simulink model "IEEE9_case"  (R2024b)
settings: Solver=FixedStepAuto  StartTime=0  StopTime=5  FixedStep=1e-7  RelTol=1e-3
values from neighbouring files (symbols this model uses):
  SG_D_1_D = 0.01056    [IEEE9_case_parameters.m]    (also in case1_parameters.m; case2_parameters.m; case3_parameters.m; case4_parameters.m)
  SG_D_1_EnableSaturation = 0    [IEEE9_case_parameters.m]    (also in case1_parameters.m; case2_parameters.m; case3_parameters.m; case4_parameters.m)
  SG_D_1_f0 = 60    [IEEE9_case_parameters.m]    (also in case1_parameters.m; case2_parameters.m; case3_parameters.m; case4_parameters.m)
  SG_D_1_H = 7.5    [IEEE9_case_parameters.m]    (also in case1_parameters.m; case2_parameters.m; case3_parameters.m; case4_parameters.m)
  SG_D_1_K_A = 20    [IEEE9_case_parameters.m]    (also in case1_parameters.m; case2_parameters.m; case3_parameters.m; case4_parameters.m)
  SG_D_1_K_E = 1.000000e+1    (= 10)    [IEEE9_case_parameters.m]    (also in case1_parameters.m; case2_parameters.m; case3_parameters.m; case4_parameters.m)
  SG_D_1_K_F = 2.363    [IEEE9_case_parameters.m]    (also in case1_parameters.m; case2_parameters.m; case3_parameters.m; case4_parameters.m)
  SG_D_1_K_s = 0.5    [IEEE9_case_parameters.m]    (also in case1_parameters.m = 5; case2_parameters.m = 5; case3_parameters.m = 5; case4_parameters.m = 5)
  SG_D_1_R_a = 0.001088    [IEEE9_case_parameters.m]    (also in case1_parameters.m; case2_parameters.m; case3_parameters.m; case4_parameters.m)
  SG_D_1_S_A = 1    [IEEE9_case_parameters.m]    (also in case1_parameters.m; case2_parameters.m; case3_parameters.m; case4_parameters.m)
  SG_D_1_S_B = 0.103    [IEEE9_case_parameters.m]    (also in case1_parameters.m; case2_parameters.m; case3_parameters.m; case4_parameters.m)
  SG_D_1_S_N = 10.659857    [IEEE9_case_parameters.m]    (also in case1_parameters.m; case2_parameters.m; case3_parameters.m; case4_parameters.m)
  SG_D_1_SpeedPara = 200    [IEEE9_case_parameters.m]    (also in case1_parameters.m; case2_parameters.m; case3_parameters.m; case4_parameters.m)
  SG_D_1_T_0 = 0.720173    [IEEE9_case_parameters.m]    (also in case1_parameters.m = 0.755522; case2_parameters.m = 0.808931; case3_parameters.m = 0.869402; case4_parameters.m = 0.729316)
  SG_D_1_T_1 = 0.3    [IEEE9_case_parameters.m]    (also in case1_parameters.m; case2_parameters.m; case3_parameters.m; case4_parameters.m)
  SG_D_1_T_2 = 0.05    [IEEE9_case_parameters.m]    (also in case1_parameters.m; case2_parameters.m; case3_parameters.m; case4_parameters.m)
  SG_D_1_T_3 = 0.02    [IEEE9_case_parameters.m]    (also in case1_parameters.m; case2_parameters.m; case3_parameters.m; case4_parameters.m)
  SG_D_1_T_4 = 0.005    [IEEE9_case_parameters.m]    (also in case1_parameters.m; case2_parameters.m; case3_parameters.m; case4_parameters.m)
  SG_D_1_T_A = 0.02    [IEEE9_case_parameters.m]    (also in case1_parameters.m; case2_parameters.m; case3_parameters.m; case4_parameters.m)
  SG_D_1_T_dd = 8.000000e+0    (= 8)    [IEEE9_case_parameters.m]    (also in case1_parameters.m; case2_parameters.m; case3_parameters.m; case4_parameters.m)
  SG_D_1_T_ddd = 0.04    [IEEE9_case_parameters.m]    (also in case1_parameters.m; case2_parameters.m; case3_parameters.m; case4_parameters.m)
  SG_D_1_T_E = 0.314    [IEEE9_case_parameters.m]    (also in case1_parameters.m; case2_parameters.m; case3_parameters.m; case4_parameters.m)
  SG_D_1_T_F = 0.35    [IEEE9_case_parameters.m]    (also in case1_parameters.m; case2_parameters.m; case3_parameters.m; case4_parameters.m)
  SG_D_1_T_qd = 0.8    [IEEE9_case_parameters.m]    (also in case1_parameters.m; case2_parameters.m; case3_parameters.m; case4_parameters.m)
  SG_D_1_T_qdd = 0.02    [IEEE9_case_parameters.m]    (also in case1_parameters.m; case2_parameters.m; case3_parameters.m; case4_parameters.m)
  SG_D_1_T_speed = 0.1    [IEEE9_case_parameters.m]    (also in case1_parameters.m = 200; case2_parameters.m = 200; case3_parameters.m = 200; case4_parameters.m = 200)
  SG_D_1_T_w = 0.5    [IEEE9_case_parameters.m]    (also in case1_parameters.m; case2_parameters.m; case3_parameters.m; case4_parameters.m)
  SG_D_1_V_ref = 1.990276    [IEEE9_case_parameters.m]    (also in case1_parameters.m = 2.042296; case2_parameters.m = 2.051388; case3_parameters.m = 2.089584; case4_parameters.m = 2.01845)
  SG_D_1_w_ref = 376.991118    [IEEE9_case_parameters.m]    (also in case1_parameters.m; case2_parameters.m; case3_parameters.m; case4_parameters.m)
  SG_D_1_wb = 6.000000e+1    (= 60)    [IEEE9_case_parameters.m]    (also in case1_parameters.m; case2_parameters.m; case3_parameters.m; case4_parameters.m)
  SG_D_1_x_d = 1.9    [IEEE9_case_parameters.m]    (also in case1_parameters.m; case2_parameters.m; case3_parameters.m; case4_parameters.m)
  SG_D_1_x_dd = 0.302    [IEEE9_case_parameters.m]    (also in case1_parameters.m; case2_parameters.m; case3_parameters.m; case4_parameters.m)
  SG_D_1_x_ddd = 0.204    [IEEE9_case_parameters.m]    (also in case1_parameters.m; case2_parameters.m; case3_parameters.m; case4_parameters.m)
  SG_D_1_x_l = 0.05    [IEEE9_case_parameters.m]    (also in case1_parameters.m; case2_parameters.m; case3_parameters.m; case4_parameters.m)
  SG_D_1_x_q = 1.3    [IEEE9_case_parameters.m]    (also in case1_parameters.m; case2_parameters.m; case3_parameters.m; case4_parameters.m)
  SG_D_1_x_qd = 0.5    [IEEE9_case_parameters.m]    (also in case1_parameters.m; case2_parameters.m; case3_parameters.m; case4_parameters.m)
  SG_D_1_x_qdd = 0.3    [IEEE9_case_parameters.m]    (also in case1_parameters.m; case2_parameters.m; case3_parameters.m; case4_parameters.m)
  SG_D_2_D = 0.02    [IEEE9_case_parameters.m]    (also in case1_parameters.m; case2_parameters.m; case3_parameters.m; case4_parameters.m)
  SG_D_2_EnableSaturation = 0    [IEEE9_case_parameters.m]    (also in case1_parameters.m; case2_parameters.m; case3_parameters.m; case4_parameters.m)
  SG_D_2_f0 = 60    [IEEE9_case_parameters.m]    (also in case1_parameters.m; case2_parameters.m; case3_parameters.m; case4_parameters.m)
  SG_D_2_H = 8.000000e+0    (= 8)    [IEEE9_case_parameters.m]    (also in case1_parameters.m; case2_parameters.m; case3_parameters.m; case4_parameters.m)
  SG_D_2_K_A = 20    [IEEE9_case_parameters.m]    (also in case1_parameters.m; case2_parameters.m; case3_parameters.m; case4_parameters.m)
  SG_D_2_K_E = 1.000000e+1    (= 10)    [IEEE9_case_parameters.m]    (also in case1_parameters.m; case2_parameters.m; case3_parameters.m; case4_parameters.m)
  SG_D_2_K_F = 2.363    [IEEE9_case_parameters.m]    (also in case1_parameters.m; case2_parameters.m; case3_parameters.m; case4_parameters.m)
  SG_D_2_K_s = 0.5    [IEEE9_case_parameters.m]    (also in case1_parameters.m = 4; case2_parameters.m = 4; case3_parameters.m = 4; case4_parameters.m = 4)
  SG_D_2_R_a = 0.001088    [IEEE9_case_parameters.m]    (also in case1_parameters.m; case2_parameters.m; case3_parameters.m; case4_parameters.m)
  SG_D_2_S_A = 1    [IEEE9_case_parameters.m]    (also in case1_parameters.m; case2_parameters.m; case3_parameters.m; case4_parameters.m)
  SG_D_2_S_B = 0.103    [IEEE9_case_parameters.m]    (also in case1_parameters.m; case2_parameters.m; case3_parameters.m; case4_parameters.m)
  SG_D_2_S_N = 10.659857    [IEEE9_case_parameters.m]    (also in case1_parameters.m; case2_parameters.m; case3_parameters.m; case4_parameters.m)
  SG_D_2_SpeedPara = 200    [IEEE9_case_parameters.m]    (also in case1_parameters.m; case2_parameters.m; case3_parameters.m; case4_parameters.m)
  SG_D_2_T_0 = 1.632913    [IEEE9_case_parameters.m]    (also in case1_parameters.m = 1.632925; case2_parameters.m = 1.632915; case3_parameters.m = 1.632914; case4_parameters.m = 1.632927)
  SG_D_2_T_1 = 0.2    [IEEE9_case_parameters.m]    (also in case1_parameters.m; case2_parameters.m; case3_parameters.m; case4_parameters.m)
  SG_D_2_T_2 = 0.05    [IEEE9_case_parameters.m]    (also in case1_parameters.m; case2_parameters.m; case3_parameters.m; case4_parameters.m)
  SG_D_2_T_3 = 0.02    [IEEE9_case_parameters.m]    (also in case1_parameters.m; case2_parameters.m; case3_parameters.m; case4_parameters.m)
  SG_D_2_T_4 = 0.005    [IEEE9_case_parameters.m]    (also in case1_parameters.m; case2_parameters.m; case3_parameters.m; case4_parameters.m)
  SG_D_2_T_A = 0.02    [IEEE9_case_parameters.m]    (also in case1_parameters.m; case2_parameters.m; case3_parameters.m; case4_parameters.m)
  SG_D_2_T_dd = 7.9    [IEEE9_case_parameters.m]    (also in case1_parameters.m; case2_parameters.m; case3_parameters.m; case4_parameters.m)
  SG_D_2_T_ddd = 0.04    [IEEE9_case_parameters.m]    (also in case1_parameters.m; case2_parameters.m; case3_parameters.m; case4_parameters.m)
  SG_D_2_T_E = 0.314    [IEEE9_case_parameters.m]    (also in case1_parameters.m; case2_parameters.m; case3_parameters.m; case4_parameters.m)
  SG_D_2_T_F = 0.35    [IEEE9_case_parameters.m]    (also in case1_parameters.m; case2_parameters.m; case3_parameters.m; case4_parameters.m)
  SG_D_2_T_qd = 0.8    [IEEE9_case_parameters.m]    (also in case1_parameters.m; case2_parameters.m; case3_parameters.m; case4_parameters.m)
  SG_D_2_T_qdd = 0.015    [IEEE9_case_parameters.m]    (also in case1_parameters.m; case2_parameters.m; case3_parameters.m; case4_parameters.m)
  SG_D_2_T_speed = 0.1    [IEEE9_case_parameters.m]    (also in case1_parameters.m = 150; case2_parameters.m = 150; case3_parameters.m = 150; case4_parameters.m = 150)
  SG_D_2_T_w = 0.35    [IEEE9_case_parameters.m]    (also in case1_parameters.m; case2_parameters.m; case3_parameters.m; case4_parameters.m)
  SG_D_2_V_ref = 2.58547    [IEEE9_case_parameters.m]    (also in case1_parameters.m = 2.597896; case2_parameters.m = 2.587136; case3_parameters.m = 2.586042; case4_parameters.m = 2.599679)
  SG_D_2_w_ref = 376.991118    [IEEE9_case_parameters.m]    (also in case1_parameters.m; case2_parameters.m; case3_parameters.m; case4_parameters.m)
  SG_D_2_wb = 6.000000e+1    (= 60)    [IEEE9_case_parameters.m]    (also in case1_parameters.m; case2_parameters.m; case3_parameters.m; case4_parameters.m)
  SG_D_2_x_d = 1.8    [IEEE9_case_parameters.m]    (also in case1_parameters.m; case2_parameters.m; case3_parameters.m; case4_parameters.m)
  SG_D_2_x_dd = 0.302    [IEEE9_case_parameters.m]    (also in case1_parameters.m; case2_parameters.m; case3_parameters.m; case4_parameters.m)
  SG_D_2_x_ddd = 0.204    [IEEE9_case_parameters.m]    (also in case1_parameters.m; case2_parameters.m; case3_parameters.m; case4_parameters.m)
  SG_D_2_x_l = 0.05    [IEEE9_case_parameters.m]    (also in case1_parameters.m; case2_parameters.m; case3_parameters.m; case4_parameters.m)
  SG_D_2_x_q = 1.25    [IEEE9_case_parameters.m]    (also in case1_parameters.m; case2_parameters.m; case3_parameters.m; case4_parameters.m)
  SG_D_2_x_qd = 0.5    [IEEE9_case_parameters.m]    (also in case1_parameters.m; case2_parameters.m; case3_parameters.m; case4_parameters.m)
  SG_D_2_x_qdd = 0.3    [IEEE9_case_parameters.m]    (also in case1_parameters.m; case2_parameters.m; case3_parameters.m; case4_parameters.m)
  SG_D_3_D = 0.02    [IEEE9_case_parameters.m]    (also in case1_parameters.m; case2_parameters.m; case3_parameters.m; case4_parameters.m)
  SG_D_3_EnableSaturation = 0    [IEEE9_case_parameters.m]    (also in case1_parameters.m; case2_parameters.m; case3_parameters.m; case4_parameters.m)
  SG_D_3_f0 = 60    [IEEE9_case_parameters.m]    (also in case1_parameters.m; case2_parameters.m; case3_parameters.m; case4_parameters.m)
  SG_D_3_H = 7.7    [IEEE9_case_parameters.m]    (also in case1_parameters.m; case2_parameters.m; case3_parameters.m; case4_parameters.m)
  SG_D_3_K_A = 20    [IEEE9_case_parameters.m]    (also in case1_parameters.m; case2_parameters.m; case3_parameters.m; case4_parameters.m)
  SG_D_3_K_E = 1.000000e+1    (= 10)    [IEEE9_case_parameters.m]    (also in case1_parameters.m; case2_parameters.m; case3_parameters.m; case4_parameters.m)
  SG_D_3_K_F = 2.363    [IEEE9_case_parameters.m]    (also in case1_parameters.m; case2_parameters.m; case3_parameters.m; case4_parameters.m)
  SG_D_3_K_s = 0.2    [IEEE9_case_parameters.m]    (also in case1_parameters.m = 2; case2_parameters.m = 2; case3_parameters.m = 2; case4_parameters.m = 2)
  SG_D_3_R_a = 0.001088    [IEEE9_case_parameters.m]    (also in case1_parameters.m; case2_parameters.m; case3_parameters.m; case4_parameters.m)
  SG_D_3_S_A = 1    [IEEE9_case_parameters.m]    (also in case1_parameters.m; case2_parameters.m; case3_parameters.m; case4_parameters.m)
  SG_D_3_S_B = 0.103    [IEEE9_case_parameters.m]    (also in case1_parameters.m; case2_parameters.m; case3_parameters.m; case4_parameters.m)
  SG_D_3_S_N = 10.659857    [IEEE9_case_parameters.m]    (also in case1_parameters.m; case2_parameters.m; case3_parameters.m; case4_parameters.m)
  SG_D_3_SpeedPara = 200    [IEEE9_case_parameters.m]    (also in case1_parameters.m; case2_parameters.m; case3_parameters.m; case4_parameters.m)
  SG_D_3_T_0 = 0.850788    [IEEE9_case_parameters.m]    (also in case1_parameters.m = 0.850786; case2_parameters.m = 0.850787; case3_parameters.m; case4_parameters.m = 0.850786)
  SG_D_3_T_1 = 0.2    [IEEE9_case_parameters.m]    (also in case1_parameters.m; case2_parameters.m; case3_parameters.m; case4_parameters.m)
  SG_D_3_T_2 = 0.05    [IEEE9_case_parameters.m]    (also in case1_parameters.m; case2_parameters.m; case3_parameters.m; case4_parameters.m)
  SG_D_3_T_3 = 0.02    [IEEE9_case_parameters.m]    (also in case1_parameters.m; case2_parameters.m; case3_parameters.m; case4_parameters.m)
  SG_D_3_T_4 = 0.005    [IEEE9_case_parameters.m]    (also in case1_parameters.m; case2_parameters.m; case3_parameters.m; case4_parameters.m)
  SG_D_3_T_A = 0.02    [IEEE9_case_parameters.m]    (also in case1_parameters.m; case2_parameters.m; case3_parameters.m; case4_parameters.m)
  SG_D_3_T_dd = 8.1    [IEEE9_case_parameters.m]    (also in case1_parameters.m; case2_parameters.m; case3_parameters.m; case4_parameters.m)
  SG_D_3_T_ddd = 0.04    [IEEE9_case_parameters.m]    (also in case1_parameters.m; case2_parameters.m; case3_parameters.m; case4_parameters.m)
  SG_D_3_T_E = 0.314    [IEEE9_case_parameters.m]    (also in case1_parameters.m; case2_parameters.m; case3_parameters.m; case4_parameters.m)
  SG_D_3_T_F = 0.35    [IEEE9_case_parameters.m]    (also in case1_parameters.m; case2_parameters.m; case3_parameters.m; case4_parameters.m)
  SG_D_3_T_qd = 0.8    [IEEE9_case_parameters.m]    (also in case1_parameters.m; case2_parameters.m; case3_parameters.m; case4_parameters.m)
  SG_D_3_T_qdd = 0.015    [IEEE9_case_parameters.m]    (also in case1_parameters.m; case2_parameters.m; case3_parameters.m; case4_parameters.m)
  SG_D_3_T_speed = 0.1    [IEEE9_case_parameters.m]    (also in case1_parameters.m = 180; case2_parameters.m = 180; case3_parameters.m = 180; case4_parameters.m = 180)
  SG_D_3_T_w = 0.4    [IEEE9_case_parameters.m]    (also in case1_parameters.m; case2_parameters.m; case3_parameters.m; case4_parameters.m)
  SG_D_3_V_ref = 1.892727    [IEEE9_case_parameters.m]    (also in case1_parameters.m = 1.906439; case2_parameters.m = 1.895535; case3_parameters.m = 1.892105; case4_parameters.m = 1.906598)
  SG_D_3_w_ref = 376.991118    [IEEE9_case_parameters.m]    (also in case1_parameters.m; case2_parameters.m; case3_parameters.m; case4_parameters.m)
  SG_D_3_wb = 6.000000e+1    (= 60)    [IEEE9_case_parameters.m]    (also in case1_parameters.m; case2_parameters.m; case3_parameters.m; case4_parameters.m)
  SG_D_3_x_d = 1.85    [IEEE9_case_parameters.m]    (also in case1_parameters.m; case2_parameters.m; case3_parameters.m; case4_parameters.m)
  SG_D_3_x_dd = 0.302    [IEEE9_case_parameters.m]    (also in case1_parameters.m; case2_parameters.m; case3_parameters.m; case4_parameters.m)
  SG_D_3_x_ddd = 0.204    [IEEE9_case_parameters.m]    (also in case1_parameters.m; case2_parameters.m; case3_parameters.m; case4_parameters.m)
  SG_D_3_x_l = 0.05    [IEEE9_case_parameters.m]    (also in case1_parameters.m; case2_parameters.m; case3_parameters.m; case4_parameters.m)
  SG_D_3_x_q = 1.2    [IEEE9_case_parameters.m]    (also in case1_parameters.m; case2_parameters.m; case3_parameters.m; case4_parameters.m)
  SG_D_3_x_qd = 0.5    [IEEE9_case_parameters.m]    (also in case1_parameters.m; case2_parameters.m; case3_parameters.m; case4_parameters.m)
  SG_D_3_x_qdd = 0.3    [IEEE9_case_parameters.m]    (also in case1_parameters.m; case2_parameters.m; case3_parameters.m; case4_parameters.m)
(part 5 of 12)

== system IEEE9_case/SG_D_1/d_T_m_SG_D_1_block ==
  note: d_T_m_SG_D_1 in IEEE9_case
      | $-\frac{T_{m,\mathrm{SG},D,1}-T_{0}+\frac{\mathrm{SpeedPara}\,\left(w_{\mathrm{SG},D,1}-w_{\mathrm{ref}}\right)}{2\,f_{0}\,\pi }}{T_{\mathrm{speed}}}$
      | Automatically generated on 2025-11-01 08:47:56 .
  State_w_SG_D_1_89d82 : Inport
  State_T_m_SG_D_1_3bd62 : Inport  Port=2
  Add_715b3 : Sum
  Add_aebef : Sum
  Constant_-1_8f139 : Constant  Value=-1
  Constant_2.0_a6cee : Constant  Value=2.0
  Constant_SpeedPara_ed1d2 : Constant  Value=SpeedPara
  Constant_T_0_18144 : Constant  Value=T_0
  Constant_T_speed_88170 : Constant  Value=T_speed
  Constant_f0_4eb3d : Constant  Value=f0
  Constant_pi_29ae0 : Constant  Value=pi
  Constant_w_ref_c58c4 : Constant  Value=w_ref
  Divide_01a85 : Product  Inputs=*/
  Divide_8a74a : Product  Inputs=*/
  Product_58145 : Product
  Product_9a8d8 : Product
  Product_e1fd7 : Product
  Product_e92fd : Product
  Subtract_2de0b : Sum  Inputs=+-
  Blockout_d_T_m_SG_D_1_8e6e4 : Outport
  wires:
  Constant_-1_8f139/1 -> Product_9a8d8/1
  Constant_w_ref_c58c4/1 -> Add_aebef/2
  State_w_SG_D_1_89d82/1 -> Product_9a8d8/2
  Add_715b3/1 -> Subtract_2de0b/1
  Add_aebef/1 -> Product_e1fd7/2
  Product_9a8d8/1 -> Add_aebef/1
  Constant_2.0_a6cee/1 -> Product_e92fd/1
  Constant_pi_29ae0/1 -> Product_e92fd/2
  Constant_SpeedPara_ed1d2/1 -> Product_e1fd7/1
  Product_e92fd/1 -> Product_58145/1
  Constant_f0_4eb3d/1 -> Product_58145/2
  Constant_T_speed_88170/1 -> Divide_01a85/2
  Product_e1fd7/1 -> Divide_8a74a/1
  Product_58145/1 -> Divide_8a74a/2
  Divide_8a74a/1 -> Add_715b3/1
  Constant_T_0_18144/1 -> Add_715b3/2
  State_T_m_SG_D_1_3bd62/1 -> Subtract_2de0b/2
  Subtract_2de0b/1 -> Divide_01a85/1
  Divide_01a85/1 -> Blockout_d_T_m_SG_D_1_8e6e4/1

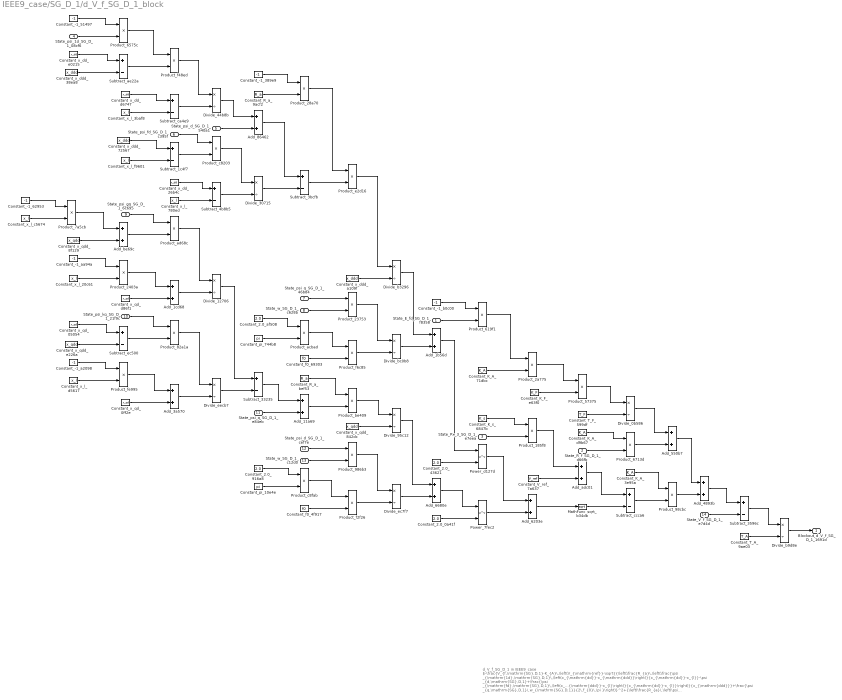
== system IEEE9_case/SG_D_1/d_V_f_SG_D_1_block ==
  note: d_V_f_SG_D_1 in IEEE9_case
      | $-\frac{V_{f,\mathrm{SG},D,1}-K_{A}\,\left(V_{\mathrm{ref}}-\sqrt{{\left(\frac{R_{a}\,\left(\frac{\psi _{\mathrm{1d},\mathrm{SG},D,1}\,\left(x_{\mathrm{dd}}-x_{\mathrm{ddd}}\right)}{x_{\mathrm{dd}}-x_{l}}-\psi _{d,\mathrm{SG},D,1}+\frac{\psi _{\mathrm{fd},\mathrm{SG},D,1}\,\left(x_{\mathrm{ddd}}-x_{l}\right)}{x_{\mathrm{dd}}-x_{l}}\right)}{x_{\mathrm{ddd}}}+\frac{\psi _{q,\mathrm{SG},D,1}\,w_{\mathrm{SG},D,1}}{2\,f_{0}\,\pi }\right)}^2+{\left(\frac{R_{a}\,\left(\psi _{q,\mathrm{SG},D,1}+\frac{\psi _{\mathrm{gq},\mathrm{SG},D,1}\,\left(x_{l}-x_{\mathrm{qdd}}\right)}{x_{l}-x_{\mathrm{qd}}}+\frac{\psi _{\mathrm{kq},\mathrm{SG},D,1}\,\left(x_{\mathrm{qd}}-x_{\mathrm{qdd}}\right)}{x_{l}-x_{\mathrm{qd}}}\right)}{x_{\mathrm{qdd}}}+\frac{\psi _{d,\mathrm{SG},D,1}\,w_{\mathrm{SG},D,1}}{2\,f_{0}\,\pi }\right)}^2}+K_{s}\,\mathrm{Px}_{3,\mathrm{SG},D,1}\right)-K_{A}\,R_{f,\mathrm{SG},D,1}+\frac{E_{\mathrm{fd},\mathrm{SG},D,1}\,K_{A}\,K_{F}}{T_{F}}}{T_{A}}$
      | Automatically generated on 2025-11-01 08:48:00 .
  State_E_fd_SG_D_1_f8358 : Inport
  State_R_f_SG_D_1_d66fb : Inport  Port=2
  State_Px_3_SG_D_1_e7eea : Inport  Port=3
  State_psi_1d_SG_D_1_08cf6 : Inport  Port=4
  State_psi_d_SG_D_1_540a1 : Inport  Port=5
  State_psi_fd_SG_D_1_c395f : Inport  Port=6
  State_psi_q_SG_D_1_46b84 : Inport  Port=7
  State_w_SG_D_1_c628b : Inport  Port=8
  State_psi_gq_SG_D_1_6c695 : Inport  Port=9
  State_psi_kq_SG_D_1_21f9c : Inport  Port=10
  State_psi_q_SG_D_1_e84eb : Inport  Port=11
  State_psi_d_SG_D_1_cef7e : Inport  Port=12
  State_w_SG_D_1_c12d0 : Inport  Port=13
  State_V_f_SG_D_1_e7d4d : Inport  Port=14
  Add_11a69 : Sum
  Add_1b56d : Sum
  Add_1cd68 : Sum
  Add_3a570 : Sum
  Add_4893b : Sum
  Add_550b7 : Sum
  Add_6203e : Sum
  Add_6680e : Sum
  Add_86462 : Sum
  Add_adc01 : Sum
  Add_be69c : Sum
  Constant_-1_389e9 : Constant  Value=-1
  Constant_-1_51497 : Constant  Value=-1
  Constant_-1_62953 : Constant  Value=-1
  Constant_-1_a2098 : Constant  Value=-1
  Constant_-1_aa94a : Constant  Value=-1
  Constant_-1_b0c00 : Constant  Value=-1
  Constant_2.0_0a41f : Constant  Value=2.0
  Constant_2.0_43621 : Constant  Value=2.0
  Constant_2.0_916a8 : Constant  Value=2.0
  Constant_2.0_af508 : Constant  Value=2.0
  Constant_K_A_3e95a : Constant  Value=K_A
  Constant_K_A_71dbc : Constant  Value=K_A
  Constant_K_A_d9b67 : Constant  Value=K_A
  Constant_K_F_e63f0 : Constant  Value=K_F
  Constant_K_s_6847b : Constant  Value=K_s
  Constant_R_a_9acf2 : Constant  Value=R_a
  Constant_R_a_bef53 : Constant  Value=R_a
  Constant_T_A_9ae03 : Constant  Value=T_A
  Constant_T_F_599df : Constant  Value=T_F
  Constant_V_ref_7a637 : Constant  Value=V_ref
  Constant_f0_4f917 : Constant  Value=f0
  Constant_f0_69303 : Constant  Value=f0
  Constant_pi_10e4e : Constant  Value=pi
  Constant_pi_744b8 : Constant  Value=pi
  Constant_x_dd_26b4c : Constant  Value=x_dd
  Constant_x_dd_d6747 : Constant  Value=x_dd
  Constant_x_dd_e0215 : Constant  Value=x_dd
  Constant_x_ddd_38ea8 : Constant  Value=x_ddd
  Constant_x_ddd_72567 : Constant  Value=x_ddd
  Constant_x_ddd_a109f : Constant  Value=x_ddd
  Constant_x_l_20c61 : Constant  Value=x_l
  Constant_x_l_3baf8 : Constant  Value=x_l
  Constant_x_l_780ed : Constant  Value=x_l
  Constant_x_l_c5674 : Constant  Value=x_l
  Constant_x_l_d5617 : Constant  Value=x_l
  Constant_x_l_f9601 : Constant  Value=x_l
  Constant_x_qd_05054 : Constant  Value=x_qd
  Constant_x_qd_0ff2e : Constant  Value=x_qd
  Constant_x_qd_d86f1 : Constant  Value=x_qd
  Constant_x_qdd_842dc : Constant  Value=x_qdd
  Constant_x_qdd_8f129 : Constant  Value=x_qdd
  Constant_x_qdd_e226a : Constant  Value=x_qdd
  Divide_0b586 : Product  Inputs=*/
  Divide_12706 : Product  Inputs=*/
  Divide_30715 : Product  Inputs=*/
  Divide_44b8b : Product  Inputs=*/
  Divide_95c12 : Product  Inputs=*/
  Divide_b3296 : Product  Inputs=*/
  Divide_b9d8e : Product  Inputs=*/
  Divide_bc0b8 : Product  Inputs=*/
  Divide_ec7f7 : Product  Inputs=*/
  Divide_eecb7 : Product  Inputs=*/
  MathFunc_sqrt_b34db : Sqrt
  Power_7fec2 : Math  Operator=pow
  Power_d127d : Math  Operator=pow
  Product_185f8 : Product
  Product_23753 : Product
  Product_2403a : Product
  Product_28a70 : Product
  Product_2a775 : Product
  Product_57375 : Product
  Product_619f1 : Product
  Product_6575c : Product
  Product_6713d : Product
  Product_7a5cb : Product
  Product_82a1a : Product
  Product_986b3 : Product
  Product_98cbc : Product
  Product_acbad : Product
  Product_ad68c : Product
  Product_be409 : Product
  Product_c8203 : Product
  Product_c8fab : Product
  Product_e2d16 : Product
  Product_f2f26 : Product
  Product_f48ed : Product
  Product_f6c85 : Product
  Product_fe995 : Product
  Subtract_1c4f7 : Sum  Inputs=+-
  Subtract_33235 : Sum  Inputs=+-
  Subtract_3596c : Sum  Inputs=+-
  Subtract_3bcfb : Sum  Inputs=+-
  Subtract_4b8b5 : Sum  Inputs=+-
  Subtract_ae22a : Sum  Inputs=+-
  Subtract_ca4e9 : Sum  Inputs=+-
  Subtract_ccca6 : Sum  Inputs=+-
  Subtract_ec500 : Sum  Inputs=+-
  Blockout_d_V_f_SG_D_1_1691d : Outport
  wires:
  Constant_-1_a2098/1 -> Product_fe995/1
  Constant_-1_62953/1 -> Product_7a5cb/1
  State_psi_d_SG_D_1_cef7e/1 -> Product_986b3/1
  Constant_x_qd_0ff2e/1 -> Add_3a570/2
  Constant_x_qdd_8f129/1 -> Add_be69c/2
  State_w_SG_D_1_c12d0/1 -> Product_986b3/2
  Constant_x_l_c5674/1 -> Product_7a5cb/2
  Subtract_3bcfb/1 -> Product_e2d16/2
  Constant_x_l_d5617/1 -> Product_fe995/2
  Constant_x_dd_e0215/1 -> Subtract_ae22a/1
  Constant_R_a_9acf2/1 -> Product_28a70/2
  Constant_-1_51497/1 -> Product_6575c/1
  Divide_30715/1 -> Subtract_3bcfb/2
  Constant_x_ddd_38ea8/1 -> Subtract_ae22a/2
  Add_3a570/1 -> Divide_eecb7/2
  State_psi_1d_SG_D_1_08cf6/1 -> Product_6575c/2
  Add_1cd68/1 -> Divide_12706/2
  Subtract_ec500/1 -> Product_82a1a/2
  Product_57375/1 -> Divide_0b586/1
  Product_acbad/1 -> Product_f6c85/1
  Product_7a5cb/1 -> Add_be69c/1
  Constant_-1_aa94a/1 -> Product_2403a/1
  Constant_x_l_20c61/1 -> Product_2403a/2
  Add_86462/1 -> Subtract_3bcfb/1
  Constant_2.0_916a8/1 -> Product_c8fab/1
  Constant_x_qd_05054/1 -> Subtract_ec500/1
  Product_6575c/1 -> Product_f48ed/1
  Constant_pi_10e4e/1 -> Product_c8fab/2
  Constant_x_qdd_e226a/1 -> Subtract_ec500/2
  Subtract_ae22a/1 -> Product_f48ed/2
  State_psi_q_SG_D_1_e84eb/1 -> Add_11a69/2
  Constant_x_dd_d6747/1 -> Subtract_ca4e9/1
  Constant_x_l_3baf8/1 -> Subtract_ca4e9/2
  Constant_x_ddd_72567/1 -> Subtract_1c4f7/1
  Constant_x_l_f9601/1 -> Subtract_1c4f7/2
  State_psi_gq_SG_D_1_6c695/1 -> Product_ad68c/1
  Add_be69c/1 -> Product_ad68c/2
  Product_2403a/1 -> Add_1cd68/1
  Constant_x_qd_d86f1/1 -> Add_1cd68/2
  Divide_44b8b/1 -> Add_86462/1
  Subtract_ca4e9/1 -> Divide_44b8b/2
  State_psi_kq_SG_D_1_21f9c/1 -> Product_82a1a/1
  Divide_b9d8e/1 -> Blockout_d_V_f_SG_D_1_1691d/1
  Product_fe995/1 -> Add_3a570/1
  Product_f48ed/1 -> Divide_44b8b/1
  State_psi_fd_SG_D_1_c395f/1 -> Product_c8203/1
  State_w_SG_D_1_c628b/1 -> Product_23753/2
  Subtract_1c4f7/1 -> Product_c8203/2
  Constant_x_dd_26b4c/1 -> Subtract_4b8b5/1
  Constant_x_l_780ed/1 -> Subtract_4b8b5/2
  Product_ad68c/1 -> Divide_12706/1
  Product_28a70/1 -> Product_e2d16/1
  Product_82a1a/1 -> Divide_eecb7/1
  State_psi_d_SG_D_1_540a1/1 -> Add_86462/2
  Product_c8203/1 -> Divide_30715/1
  Subtract_4b8b5/1 -> Divide_30715/2
  Divide_12706/1 -> Subtract_33235/1
  Divide_eecb7/1 -> Subtract_33235/2
  Constant_-1_389e9/1 -> Product_28a70/1
  Constant_2.0_af508/1 -> Product_acbad/1
  Constant_pi_744b8/1 -> Product_acbad/2
  Subtract_33235/1 -> Add_11a69/1
  State_psi_q_SG_D_1_46b84/1 -> Product_23753/1
  Constant_f0_69303/1 -> Product_f6c85/2
  Constant_R_a_bef53/1 -> Product_be409/1
  Add_11a69/1 -> Product_be409/2
  Product_c8fab/1 -> Product_f2f26/1
  Power_d127d/1 -> Add_6203e/1
  Constant_f0_4f917/1 -> Product_f2f26/2
  Product_e2d16/1 -> Divide_b3296/1
  Constant_x_ddd_a109f/1 -> Divide_b3296/2
  Product_23753/1 -> Divide_bc0b8/1
  Product_f6c85/1 -> Divide_bc0b8/2
  Product_be409/1 -> Divide_95c12/1
  Constant_x_qdd_842dc/1 -> Divide_95c12/2
  Product_986b3/1 -> Divide_ec7f7/1
  Product_f2f26/1 -> Divide_ec7f7/2
  Divide_b3296/1 -> Add_1b56d/1
  Divide_bc0b8/1 -> Add_1b56d/2
  Divide_95c12/1 -> Add_6680e/1
  Divide_ec7f7/1 -> Add_6680e/2
  Constant_-1_b0c00/1 -> Product_619f1/1
  State_E_fd_SG_D_1_f8358/1 -> Product_619f1/2
  Add_1b56d/1 -> Power_d127d/1
  Constant_2.0_43621/1 -> Power_d127d/2
  Add_6680e/1 -> Power_7fec2/1
  Constant_2.0_0a41f/1 -> Power_7fec2/2
  Product_619f1/1 -> Product_2a775/1
  Constant_K_A_71dbc/1 -> Product_2a775/2
  Constant_K_s_6847b/1 -> Product_185f8/1
  State_Px_3_SG_D_1_e7eea/1 -> Product_185f8/2
  Power_7fec2/1 -> Add_6203e/2
  Divide_0b586/1 -> Add_550b7/1
  Product_2a775/1 -> Product_57375/1
  Constant_K_F_e63f0/1 -> Product_57375/2
  Product_185f8/1 -> Add_adc01/1
  Constant_V_ref_7a637/1 -> Add_adc01/2
  Add_6203e/1 -> MathFunc_sqrt_b34db/1
  Constant_T_F_599df/1 -> Divide_0b586/2
  Constant_K_A_d9b67/1 -> Product_6713d/1
  State_R_f_SG_D_1_d66fb/1 -> Product_6713d/2
  Add_adc01/1 -> Subtract_ccca6/1
  MathFunc_sqrt_b34db/1 -> Subtract_ccca6/2
  Constant_T_A_9ae03/1 -> Divide_b9d8e/2
  Product_6713d/1 -> Add_550b7/2
  Constant_K_A_3e95a/1 -> Product_98cbc/1
  Subtract_ccca6/1 -> Product_98cbc/2
  Add_550b7/1 -> Add_4893b/1
  Product_98cbc/1 -> Add_4893b/2
  Add_4893b/1 -> Subtract_3596c/1
  State_V_f_SG_D_1_e7d4d/1 -> Subtract_3596c/2
  Subtract_3596c/1 -> Divide_b9d8e/1

== system IEEE9_case/SG_D_1/d_psi_1d_SG_D_1_block ==
  note: d_psi_1d_SG_D_1 in IEEE9_case
      | $-\frac{\psi _{\mathrm{1d},\mathrm{SG},D,1}-\psi _{\mathrm{fd},\mathrm{SG},D,1}+\frac{\left(x_{\mathrm{dd}}-x_{l}\right)\,\left(\frac{\psi _{\mathrm{1d},\mathrm{SG},D,1}\,\left(x_{\mathrm{dd}}-x_{\mathrm{ddd}}\right)}{x_{\mathrm{dd}}-x_{l}}-\psi _{d,\mathrm{SG},D,1}+\frac{\psi _{\mathrm{fd},\mathrm{SG},D,1}\,\left(x_{\mathrm{ddd}}-x_{l}\right)}{x_{\mathrm{dd}}-x_{l}}\right)}{x_{\mathrm{ddd}}}}{T_{\mathrm{ddd}}}$
      | Automatically generated on 2025-11-01 08:47:38 .
  State_psi_1d_SG_D_1_7d745 : Inport
  State_psi_fd_SG_D_1_7c5ea : Inport  Port=2
  State_psi_1d_SG_D_1_1205e : Inport  Port=3
  State_psi_d_SG_D_1_3c3e9 : Inport  Port=4
  State_psi_fd_SG_D_1_d1f9e : Inport  Port=5
  Add_298d0 : Sum
  Add_ae5fc : Sum
  Add_e105b : Sum
  Constant_-1_85f80 : Constant  Value=-1
  Constant_-1_ac343 : Constant  Value=-1
  Constant_T_ddd_f4225 : Constant  Value=T_ddd
  Constant_x_dd_4005e : Constant  Value=x_dd
  Constant_x_dd_65a07 : Constant  Value=x_dd
  Constant_x_dd_737f8 : Constant  Value=x_dd
  Constant_x_dd_bbdd7 : Constant  Value=x_dd
  Constant_x_ddd_9f231 : Constant  Value=x_ddd
  Constant_x_ddd_a7848 : Constant  Value=x_ddd
  Constant_x_ddd_b2df7 : Constant  Value=x_ddd
  Constant_x_l_47893 : Constant  Value=x_l
  Constant_x_l_76afa : Constant  Value=x_l
  Constant_x_l_b838e : Constant  Value=x_l
  Constant_x_l_d5dc8 : Constant  Value=x_l
  Divide_888c1 : Product  Inputs=*/
  Divide_94e88 : Product  Inputs=*/
  Divide_ef831 : Product  Inputs=*/
  Divide_faa1f : Product  Inputs=*/
  Product_01b00 : Product
  Product_471e7 : Product
  Product_50cf9 : Product
  Product_9b48e : Product
  Product_e113d : Product
  Subtract_69a33 : Sum  Inputs=+-
  Subtract_7e7d6 : Sum  Inputs=+-
  Subtract_88e6d : Sum  Inputs=+-
  Subtract_b4855 : Sum  Inputs=+-
  Subtract_c042c : Sum  Inputs=+-
  Subtract_f8307 : Sum  Inputs=+-
  Blockout_d_psi_1d_SG_D_1_c59e9 : Outport
  wires:
  Product_471e7/1 -> Product_9b48e/1
  Constant_-1_ac343/1 -> Product_471e7/1
  Subtract_7e7d6/1 -> Product_9b48e/2
  State_psi_1d_SG_D_1_1205e/1 -> Product_471e7/2
  Subtract_69a33/1 -> Product_e113d/1
  State_psi_d_SG_D_1_3c3e9/1 -> Add_ae5fc/2
  Constant_x_dd_4005e/1 -> Subtract_f8307/1
  Constant_x_l_76afa/1 -> Subtract_69a33/2
  Constant_x_dd_65a07/1 -> Subtract_7e7d6/1
  Subtract_88e6d/1 -> Product_50cf9/2
  Constant_x_l_47893/1 -> Subtract_f8307/2
  Divide_888c1/1 -> Subtract_c042c/2
  Constant_x_ddd_9f231/1 -> Subtract_7e7d6/2
  Constant_x_ddd_b2df7/1 -> Subtract_88e6d/1
  Constant_x_l_d5dc8/1 -> Subtract_88e6d/2
  Add_e105b/1 -> Add_298d0/1
  Product_9b48e/1 -> Divide_faa1f/1
  Divide_ef831/1 -> Add_298d0/2
  Subtract_f8307/1 -> Divide_faa1f/2
  State_psi_fd_SG_D_1_d1f9e/1 -> Product_50cf9/1
  Constant_x_dd_bbdd7/1 -> Subtract_b4855/1
  Constant_x_l_b838e/1 -> Subtract_b4855/2
  Constant_x_ddd_a7848/1 -> Divide_ef831/2
  Subtract_c042c/1 -> Product_e113d/2
  Divide_faa1f/1 -> Add_ae5fc/1
  Product_50cf9/1 -> Divide_888c1/1
  Subtract_b4855/1 -> Divide_888c1/2
  Product_e113d/1 -> Divide_ef831/1
  Constant_x_dd_737f8/1 -> Subtract_69a33/1
  Add_ae5fc/1 -> Subtract_c042c/1
  Constant_-1_85f80/1 -> Product_01b00/1
  State_psi_1d_SG_D_1_7d745/1 -> Product_01b00/2
  Product_01b00/1 -> Add_e105b/1
  State_psi_fd_SG_D_1_7c5ea/1 -> Add_e105b/2
  Add_298d0/1 -> Divide_94e88/1
  Constant_T_ddd_f4225/1 -> Divide_94e88/2
  Divide_94e88/1 -> Blockout_d_psi_1d_SG_D_1_c59e9/1

== system IEEE9_case/SG_D_1/d_psi_d_SG_D_1_block ==
  note: d_psi_d_SG_D_1 in IEEE9_case
      | $2\,\pi \,f_{0}\,\left(v_{d,\mathrm{SG},D,1}\,\sin\left(\theta _{\mathrm{SG},D,1}\right)-v_{q,\mathrm{SG},D,1}\,\cos\left(\theta _{\mathrm{SG},D,1}\right)+\frac{R_{a}\,\left(\frac{\psi _{\mathrm{1d},\mathrm{SG},D,1}\,\left(x_{\mathrm{dd}}-x_{\mathrm{ddd}}\right)}{x_{\mathrm{dd}}-x_{l}}-\psi _{d,\mathrm{SG},D,1}+\frac{\psi _{\mathrm{fd},\mathrm{SG},D,1}\,\left(x_{\mathrm{ddd}}-x_{l}\right)}{x_{\mathrm{dd}}-x_{l}}\right)}{x_{\mathrm{ddd}}}+\frac{\psi _{q,\mathrm{SG},D,1}\,w_{\mathrm{SG},D,1}}{2\,f_{0}\,\pi }\right)$
      | Automatically generated on 2025-11-01 08:47:24 .
  State_psi_1d_SG_D_1_1f550 : Inport
  State_psi_d_SG_D_1_ce2c6 : Inport  Port=2
  State_psi_fd_SG_D_1_3d49f : Inport  Port=3
  Input_v_d_SG_D_1_42b00 : Inport  Port=4
  State_theta_SG_D_1_3952e : Inport  Port=5
  Input_v_q_SG_D_1_ee29c : Inport  Port=6
  State_theta_SG_D_1_113de : Inport  Port=7
  State_psi_q_SG_D_1_72117 : Inport  Port=8
  State_w_SG_D_1_6f6c4 : Inport  Port=9
  Add_4cb4b : Sum
  Add_f6153 : Sum
  Constant_-1_c1a33 : Constant  Value=-1
  Constant_-2.0_56455 : Constant  Value=-2.0
  Constant_2.0_358eb : Constant  Value=2.0
  Constant_R_a_48f89 : Constant  Value=R_a
  Constant_f0_145c8 : Constant  Value=f0
  Constant_f0_c4db2 : Constant  Value=f0
  Constant_pi_394fc : Constant  Value=pi
  Constant_pi_8c389 : Constant  Value=pi
  Constant_x_dd_16684 : Constant  Value=x_dd
  Constant_x_dd_9ac76 : Constant  Value=x_dd
  Constant_x_dd_e96b3 : Constant  Value=x_dd
  Constant_x_ddd_52b06 : Constant  Value=x_ddd
  Constant_x_ddd_9b69e : Constant  Value=x_ddd
  Constant_x_ddd_a5c8c : Constant  Value=x_ddd
  Constant_x_l_32f3a : Constant  Value=x_l
  Constant_x_l_d2a98 : Constant  Value=x_l
  Constant_x_l_d2c26 : Constant  Value=x_l
  Divide_4033e : Product  Inputs=*/
  Divide_ad9dd : Product  Inputs=*/
  Divide_ed241 : Product  Inputs=*/
  Divide_ee7c5 : Product  Inputs=*/
  MathFunc_cos_e01cf : Trigonometry  Operator=cos
  MathFunc_sin_e5a5e : Trigonometry
  Product_24ad3 : Product
  Product_2b527 : Product
  Product_312bb : Product
  Product_39ba4 : Product
  Product_5f269 : Product
  Product_68a16 : Product
  Product_77e24 : Product
  Product_87a2c : Product
  Product_9a0e2 : Product
  Product_b0706 : Product
  Product_c67ab : Product
  Product_e05cb : Product
  Subtract_64213 : Sum  Inputs=+-
  Subtract_644a3 : Sum  Inputs=+-
  Subtract_be21d : Sum  Inputs=+-
  Subtract_c34bd : Sum  Inputs=+-
  Subtract_cee64 : Sum  Inputs=+-
  Subtract_cf6d5 : Sum  Inputs=+-
  Subtract_f700c : Sum  Inputs=+-
  Blockout_d_psi_d_SG_D_1_736fa : Outport
  wires:
  Add_4cb4b/1 -> Subtract_c34bd/1
  Product_24ad3/1 -> Divide_ee7c5/1
  Subtract_f700c/1 -> Product_24ad3/2
  Divide_ee7c5/1 -> Add_4cb4b/1
  Product_77e24/1 -> Product_24ad3/1
  Constant_x_ddd_9b69e/1 -> Subtract_f700c/2
  Constant_x_dd_9ac76/1 -> Subtract_f700c/1
  State_psi_1d_SG_D_1_1f550/1 -> Product_77e24/2
  Constant_-1_c1a33/1 -> Product_77e24/1
  Product_68a16/1 -> Divide_4033e/1
  Constant_x_l_d2a98/1 -> Subtract_644a3/2
  State_psi_d_SG_D_1_ce2c6/1 -> Add_4cb4b/2
  Constant_x_dd_e96b3/1 -> Subtract_644a3/1
  Constant_x_ddd_a5c8c/1 -> Subtract_64213/1
  Constant_x_l_d2c26/1 -> Subtract_64213/2
  Subtract_644a3/1 -> Divide_ee7c5/2
  State_psi_fd_SG_D_1_3d49f/1 -> Product_68a16/1
  Constant_x_ddd_52b06/1 -> Divide_ad9dd/2
  Subtract_64213/1 -> Product_68a16/2
  Product_9a0e2/1 -> Subtract_cee64/2
  Constant_x_dd_16684/1 -> Subtract_cf6d5/1
  Constant_x_l_32f3a/1 -> Subtract_cf6d5/2
  Subtract_cf6d5/1 -> Divide_4033e/2
  Divide_4033e/1 -> Subtract_c34bd/2
  Constant_R_a_48f89/1 -> Product_b0706/1
  Subtract_c34bd/1 -> Product_b0706/2
  MathFunc_cos_e01cf/1 -> Product_e05cb/2
  State_theta_SG_D_1_3952e/1 -> MathFunc_sin_e5a5e/1
  Divide_ad9dd/1 -> Subtract_cee64/1
  Product_b0706/1 -> Divide_ad9dd/1
  MathFunc_sin_e5a5e/1 -> Product_9a0e2/2
  Input_v_d_SG_D_1_42b00/1 -> Product_9a0e2/1
  Product_87a2c/1 -> Blockout_d_psi_d_SG_D_1_736fa/1
  Product_312bb/1 -> Product_87a2c/1
  Product_5f269/1 -> Product_312bb/1
  State_theta_SG_D_1_113de/1 -> MathFunc_cos_e01cf/1
  Constant_2.0_358eb/1 -> Product_39ba4/1
  Constant_pi_394fc/1 -> Product_39ba4/2
  Input_v_q_SG_D_1_ee29c/1 -> Product_e05cb/1
  Constant_f0_c4db2/1 -> Product_312bb/2
  State_psi_q_SG_D_1_72117/1 -> Product_c67ab/1
  State_w_SG_D_1_6f6c4/1 -> Product_c67ab/2
  Product_39ba4/1 -> Product_2b527/1
  Constant_pi_8c389/1 -> Product_5f269/2
  Constant_f0_145c8/1 -> Product_2b527/2
  Constant_-2.0_56455/1 -> Product_5f269/1
  Add_f6153/1 -> Subtract_be21d/1
  Subtract_cee64/1 -> Add_f6153/1
  Product_e05cb/1 -> Add_f6153/2
  Product_c67ab/1 -> Divide_ed241/1
  Product_2b527/1 -> Divide_ed241/2
  Divide_ed241/1 -> Subtract_be21d/2
  Subtract_be21d/1 -> Product_87a2c/2

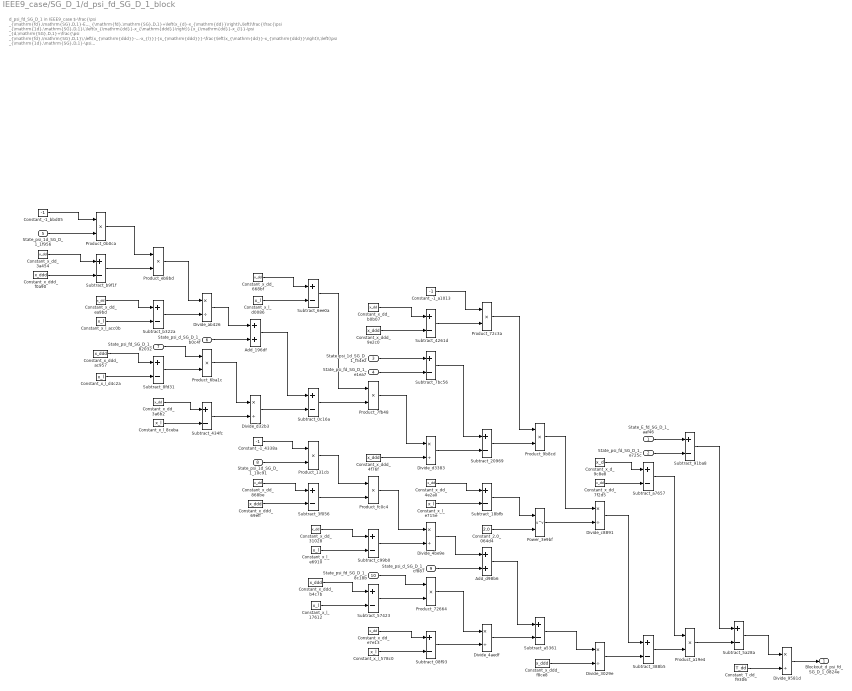
== system IEEE9_case/SG_D_1/d_psi_fd_SG_D_1_block ==
  note: d_psi_fd_SG_D_1 in IEEE9_case
      | $-\frac{\psi _{\mathrm{fd},\mathrm{SG},D,1}-E_{\mathrm{fd},\mathrm{SG},D,1}+\left(x_{d}-x_{\mathrm{dd}}\right)\,\left(\frac{\frac{\psi _{\mathrm{1d},\mathrm{SG},D,1}\,\left(x_{\mathrm{dd}}-x_{\mathrm{ddd}}\right)}{x_{\mathrm{dd}}-x_{l}}-\psi _{d,\mathrm{SG},D,1}+\frac{\psi _{\mathrm{fd},\mathrm{SG},D,1}\,\left(x_{\mathrm{ddd}}-x_{l}\right)}{x_{\mathrm{dd}}-x_{l}}}{x_{\mathrm{ddd}}}-\frac{\left(x_{\mathrm{dd}}-x_{\mathrm{ddd}}\right)\,\left(\psi _{\mathrm{1d},\mathrm{SG},D,1}-\psi _{\mathrm{fd},\mathrm{SG},D,1}+\frac{\left(x_{\mathrm{dd}}-x_{l}\right)\,\left(\frac{\psi _{\mathrm{1d},\mathrm{SG},D,1}\,\left(x_{\mathrm{dd}}-x_{\mathrm{ddd}}\right)}{x_{\mathrm{dd}}-x_{l}}-\psi _{d,\mathrm{SG},D,1}+\frac{\psi _{\mathrm{fd},\mathrm{SG},D,1}\,\left(x_{\mathrm{ddd}}-x_{l}\right)}{x_{\mathrm{dd}}-x_{l}}\right)}{x_{\mathrm{ddd}}}\right)}{{\left(x_{\mathrm{dd}}-x_{l}\right)}^2}\right)}{T_{\mathrm{dd}}}$
      | Automatically generated on 2025-11-01 08:47:35 .
  State_E_fd_SG_D_1_aaf46 : Inport
  State_psi_fd_SG_D_1_e725c : Inport  Port=2
  State_psi_1d_SG_D_1_f54e2 : Inport  Port=3
  State_psi_fd_SG_D_1_e1ea7 : Inport  Port=4
  State_psi_1d_SG_D_1_1f956 : Inport  Port=5
  State_psi_d_SG_D_1_b0c4f : Inport  Port=6
  State_psi_fd_SG_D_1_82032 : Inport  Port=7
  State_psi_1d_SG_D_1_10c91 : Inport  Port=8
  State_psi_d_SG_D_1_cf887 : Inport  Port=9
  State_psi_fd_SG_D_1_8c18b : Inport  Port=10
  Add_196df : Sum
  Add_d98b6 : Sum
  Constant_-1_4338a : Constant  Value=-1
  Constant_-1_a1013 : Constant  Value=-1
  Constant_-1_bbd05 : Constant  Value=-1
  Constant_2.0_064d4 : Constant  Value=2.0
  Constant_T_dd_f9306 : Constant  Value=T_dd
  Constant_x_d_9c8e8 : Constant  Value=x_d
  Constant_x_dd_31028 : Constant  Value=x_dd
  Constant_x_dd_3a454 : Constant  Value=x_dd
  Constant_x_dd_3a6b2 : Constant  Value=x_dd
  Constant_x_dd_4e2a0 : Constant  Value=x_dd
  Constant_x_dd_668bf : Constant  Value=x_dd
  Constant_x_dd_7f2d5 : Constant  Value=x_dd
  Constant_x_dd_868be : Constant  Value=x_dd
  Constant_x_dd_b0b07 : Constant  Value=x_dd
  Constant_x_dd_e7e13 : Constant  Value=x_dd
  Constant_x_dd_ea9bd : Constant  Value=x_dd
  Constant_x_ddd_4f76f : Constant  Value=x_ddd
  Constant_x_ddd_69eff : Constant  Value=x_ddd
  Constant_x_ddd_9e2c0 : Constant  Value=x_ddd
  Constant_x_ddd_ac957 : Constant  Value=x_ddd
  Constant_x_ddd_b4c7b : Constant  Value=x_ddd
  Constant_x_ddd_f0a90 : Constant  Value=x_ddd
  Constant_x_ddd_f8ce8 : Constant  Value=x_ddd
  Constant_x_l_17612 : Constant  Value=x_l
  Constant_x_l_578c0 : Constant  Value=x_l
  Constant_x_l_8ceba : Constant  Value=x_l
  Constant_x_l_acc0b : Constant  Value=x_l
  Constant_x_l_d0086 : Constant  Value=x_l
  Constant_x_l_d4c2a : Constant  Value=x_l
  Constant_x_l_e6910 : Constant  Value=x_l
  Constant_x_l_e715e : Constant  Value=x_l
  Divide_3029e : Product  Inputs=*/
  Divide_4aedf : Product  Inputs=*/
  Divide_4be9e : Product  Inputs=*/
  Divide_9581d : Product  Inputs=*/
  Divide_ab426 : Product  Inputs=*/
  Divide_c8891 : Product  Inputs=*/
  Divide_d32b3 : Product  Inputs=*/
  Divide_d3383 : Product  Inputs=*/
  Power_3e9bf : Math  Operator=pow
  Product_0b0ca : Product
  Product_131cb : Product
  Product_6ba1c : Product
  Product_72664 : Product
  Product_72c3a : Product
  Product_7fb48 : Product
  Product_9b8cd : Product
  Product_a19e4 : Product
  Product_eb8bd : Product
  Product_fc0c4 : Product
  Subtract_08f93 : Sum  Inputs=+-
  Subtract_0c16a : Sum  Inputs=+-
  Subtract_18bfb : Sum  Inputs=+-
  Subtract_20969 : Sum  Inputs=+-
  Subtract_388b5 : Sum  Inputs=+-
  Subtract_3f056 : Sum  Inputs=+-
  Subtract_4261d : Sum  Inputs=+-
  Subtract_434fc : Sum  Inputs=+-
  Subtract_57423 : Sum  Inputs=+-
  Subtract_5a28a : Sum  Inputs=+-
  Subtract_6ee0a : Sum  Inputs=+-
  Subtract_7bc56 : Sum  Inputs=+-
  Subtract_8fd31 : Sum  Inputs=+-
  Subtract_91ba8 : Sum  Inputs=+-
  Subtract_a5361 : Sum  Inputs=+-
  Subtract_a7657 : Sum  Inputs=+-
  Subtract_b322a : Sum  Inputs=+-
  Subtract_b9f1f : Sum  Inputs=+-
  Subtract_c99b0 : Sum  Inputs=+-
  Blockout_d_psi_fd_SG_D_1_0824e : Outport
  wires:
  State_psi_d_SG_D_1_b0c4f/1 -> Add_196df/2
  Constant_x_dd_ea9bd/1 -> Subtract_b322a/1
  Product_eb8bd/1 -> Divide_ab426/1
  Subtract_b9f1f/1 -> Product_eb8bd/2
  Subtract_0c16a/1 -> Product_7fb48/2
  Product_0b0ca/1 -> Product_eb8bd/1
  Constant_x_dd_3a454/1 -> Subtract_b9f1f/1
  Constant_x_l_d0086/1 -> Subtract_6ee0a/2
  Constant_-1_bbd05/1 -> Product_0b0ca/1
  Subtract_6ee0a/1 -> Product_7fb48/1
  Constant_x_l_acc0b/1 -> Subtract_b322a/2
  Constant_x_ddd_f0a90/1 -> Subtract_b9f1f/2
  State_psi_1d_SG_D_1_1f956/1 -> Product_0b0ca/2
  Constant_x_ddd_ac957/1 -> Subtract_8fd31/1
  Constant_x_l_d4c2a/1 -> Subtract_8fd31/2
  State_E_fd_SG_D_1_aaf46/1 -> Subtract_91ba8/1
  Divide_ab426/1 -> Add_196df/1
  Subtract_b322a/1 -> Divide_ab426/2
  State_psi_fd_SG_D_1_82032/1 -> Product_6ba1c/1
  Constant_x_ddd_4f76f/1 -> Divide_d3383/2
  Subtract_8fd31/1 -> Product_6ba1c/2
  Constant_x_dd_3a6b2/1 -> Subtract_434fc/1
  Constant_x_dd_4e2a0/1 -> Subtract_18bfb/1
  State_psi_fd_SG_D_1_e725c/1 -> Subtract_91ba8/2
  Constant_x_l_8ceba/1 -> Subtract_434fc/2
  Product_6ba1c/1 -> Divide_d32b3/1
  Constant_-1_a1013/1 -> Product_72c3a/1
  Subtract_434fc/1 -> Divide_d32b3/2
  Constant_x_dd_668bf/1 -> Subtract_6ee0a/1
  Add_196df/1 -> Subtract_0c16a/1
  Constant_x_l_e715e/1 -> Subtract_18bfb/2
  Divide_d32b3/1 -> Subtract_0c16a/2
  Divide_c8891/1 -> Subtract_388b5/1
  Constant_-1_4338a/1 -> Product_131cb/1
  State_psi_1d_SG_D_1_10c91/1 -> Product_131cb/2
  Constant_x_dd_868be/1 -> Subtract_3f056/1
  Subtract_4261d/1 -> Product_72c3a/2
  Constant_x_ddd_69eff/1 -> Subtract_3f056/2
  Product_131cb/1 -> Product_fc0c4/1
  Constant_2.0_064d4/1 -> Power_3e9bf/2
  Product_fc0c4/1 -> Divide_4be9e/1
  Subtract_388b5/1 -> Product_a19e4/2
  Subtract_3f056/1 -> Product_fc0c4/2
  State_psi_d_SG_D_1_cf887/1 -> Add_d98b6/2
  Constant_x_dd_31028/1 -> Subtract_c99b0/1
  Constant_x_l_e6910/1 -> Subtract_c99b0/2
  Constant_x_dd_b0b07/1 -> Subtract_4261d/1
  Divide_d3383/1 -> Subtract_20969/2
  Constant_x_ddd_b4c7b/1 -> Subtract_57423/1
  Constant_x_ddd_9e2c0/1 -> Subtract_4261d/2
  Constant_x_l_17612/1 -> Subtract_57423/2
  Subtract_57423/1 -> Product_72664/2
  State_psi_1d_SG_D_1_f54e2/1 -> Subtract_7bc56/1
  Product_72664/1 -> Divide_4aedf/1
  State_psi_fd_SG_D_1_e1ea7/1 -> Subtract_7bc56/2
  State_psi_fd_SG_D_1_8c18b/1 -> Product_72664/1
  Product_7fb48/1 -> Divide_d3383/1
  Divide_4be9e/1 -> Add_d98b6/1
  Subtract_c99b0/1 -> Divide_4be9e/2
  Constant_x_dd_e7e13/1 -> Subtract_08f93/1
  Constant_x_l_578c0/1 -> Subtract_08f93/2
  Divide_4aedf/1 -> Subtract_a5361/2
  Subtract_7bc56/1 -> Subtract_20969/1
  Subtract_08f93/1 -> Divide_4aedf/2
  Subtract_20969/1 -> Product_9b8cd/2
  Product_72c3a/1 -> Product_9b8cd/1
  Subtract_18bfb/1 -> Power_3e9bf/1
  Add_d98b6/1 -> Subtract_a5361/1
  Product_9b8cd/1 -> Divide_c8891/1
  Power_3e9bf/1 -> Divide_c8891/2
  Subtract_a5361/1 -> Divide_3029e/1
  Constant_x_ddd_f8ce8/1 -> Divide_3029e/2
  Constant_x_d_9c8e8/1 -> Subtract_a7657/1
  Constant_x_dd_7f2d5/1 -> Subtract_a7657/2
  Divide_3029e/1 -> Subtract_388b5/2
  Subtract_a7657/1 -> Product_a19e4/1
  Subtract_91ba8/1 -> Subtract_5a28a/1
  Product_a19e4/1 -> Subtract_5a28a/2
  Subtract_5a28a/1 -> Divide_9581d/1
  Constant_T_dd_f9306/1 -> Divide_9581d/2
  Divide_9581d/1 -> Blockout_d_psi_fd_SG_D_1_0824e/1
